simulink model "model2_cm"  (R2018b)
settings: Solver=ode8  StartTime=0.0  StopTime=Inf  FixedStep=0.01  RelTol=1e-3  EnableMultiTasking=on
StopFcn:
  | stopCallback
undefined symbols (not defined in the file): ipaddr, params, PTP
libraries: slrtlib x7, xpcutilitieslib x3, ptplib x3, xpcrtudplib x3, controllers_cl x1, find6DOF_cl x1, find6DOFSnell_cl x1, find6DOFSnellMin_cl x1, risingDebounce_ul x1, latchHigh_ul x1, manualMotorOverride_ul x1, outputCommands_ul x1
settings Model: sg_rtwmakecfg_data=_sglibc_  SimulationMode=external  Creator=mcobb  LastModifiedBy=MAE-NCSUCORE
settings SolverCC: ConcurrentTasks=on  AutoInsertRateTranBlk=on
settings DataIOCC: SaveFormat=StructureWithTime
settings OptimizationCC: BlockReduction=off  UseFloatMulNetSlope=on  EnhancedBackFolding=on  PassReuseOutputArgsThreshold=0  EfficientFloat2IntCast=on  OptimizeBlockOrder=speed  DifferentSizesBufferReuse=on  OptimizationCustomize=off
settings DebuggingCC: ParameterOverflowMsg=none  ParameterTunabilityLossMsg=error  LibraryContextMissingDiagnostic=none
settings HardwareCC: ProdBitPerPointer=32  ProdBitPerSizeT=32  ProdBitPerPtrDiffT=32  ProdLargestAtomicFloat=None  ProdWordSize=32  ProdLongLongMode=on  ProdHWDeviceType=Generic->32-bit x86 compatible
settings SFSimCC: SimUseLocalCustomCode=off  MATLABDynamicMemAlloc=off
settings RTWCC: SystemTargetFile=slrt.tlc  TemplateMakefile=slrt_default_tmf  Description=Simulink Real-Time  RTWUseLocalCustomCode=off  BuildConfiguration=Debug  CodeExecutionProfiling=on  RTWCompilerOptimization=on
settings CodeAppCC: ForceParamTrailComments=on  OperatorAnnotations=on
settings SimulinkRealTimeCC: SupportVariableSizeSignals=on  PreserveStateflowLocalDataDimensions=off  RL32LogTETModifier=off  RL32ObjectName=tg2  xPCisDefaultEnv=off  xPCTargetPCEnvName=Machine2  xPCConcurrentTasks=on

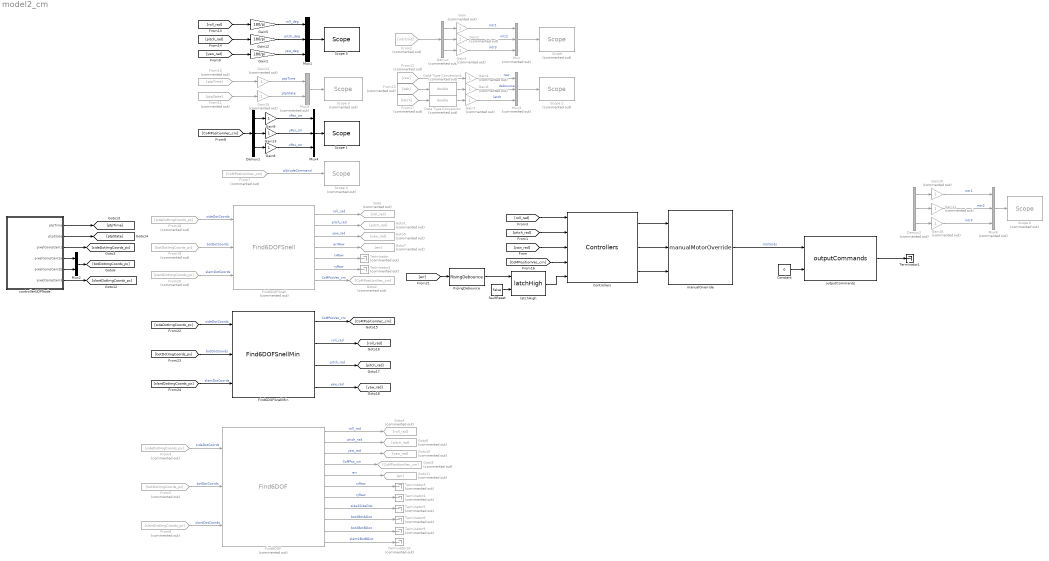
== system model2_cm ==
  Constant : Constant  Value=0
  Controllers : controllers_cl/Controllers  SystemSampleTime=-1
      link override ConstantSetpoints/AltitudeController: enable=off  kp=0.1  kd=0  timeConstant_s=0.4
      link override ConstantSetpoints/AltitudeSetpoint_cm: Value=46
      link override ConstantSetpoints/PitchController: enable=off  kp=2  kd=1  timeConstant_s=0.3
      link override ConstantSetpoints/PitchSetpoint_deg: Value=5
      link override ConstantSetpoints/RollController: enable=off  kp=2  kd=1  timeConstant_s=0.02
      link override ConstantSetpoints/RollSetpoint_deg: Value=0
  Data Type Conversion : DataTypeConversion  Commented=on  OutDataTypeStr=double
  Data Type Conversion1 : DataTypeConversion  Commented=on  OutDataTypeStr=double
  Demux : Demux  Commented=on  Outputs=3
  Demux1 : Demux  Outputs=3
  Demux2 : Demux  Commented=on  Outputs=3
  Find6DOF : find6DOF_cl/Find6DOF  Commented=on  imageDims_px=params.sideImageSize_px.Value  initialCoMPositionVec_cm=params.initCoMPosVec_cm.Value  cameraFOVAngles_deg=params.cameraFOV_deg.Value  sideEulerAngles_deg=params.sideCamEulAng_deg.Value  sideCamPositionVec_cm=params.sideCamPosVec_cm.Value  botEulerAngles_deg=params.botCamEulAng_deg.Value  botCamPositionVec_cm=params.botCamPosVec_cm.Value  slantEulerAngles_deg=params.slntCamEulAng_deg.Value  slantCamPositionVec_cm=params.slntCamPosVec_cm.Value  sideSeparation_cm=params.sideDotSepDist_cm.Value  sidePositionVecBF_cm=params.sideDotPosVec_cm.Value  bottomASeparation_cm=params.botADotSepDist_cm.Value  botAPositionVecBF_cm=params.botADotPosVec_cm.Value  bottomBSeparation_cm=params.botBDotSepDist_cm.Value  botBPositionVecBG_cm=params.botBDotPosVec_cm.Value
  Find6DOFSnell : find6DOFSnell_cl/Find6DOFSnell  Commented=on  imageDims_px=params.sideImageSize_px.Value  initialCoMPositionVec_cm=params.initCoMPosVec_cm.Value  indxOfRefVec=params.indexOfRefractionA.Value  glassThickness_cm=params.glassThickness_cm.Value  cameraFOVAngles_deg=params.cameraFOV_deg.Value  sideEulerAngles_deg=params.sideCamEulAng_deg.Value  sideCamPositionVec_cm=params.sideCamPosVec_cm.Value  sideCamDistToGlass_cm=params.sideDistancetoGlass_cm.Value  botEulerAngles_deg=params.botCamEulAng_deg.Value  botCamPositionVec_cm=params.botCamPosVec_cm.Value  botCamDistToGlass_cm=params.botDistancetoGlass_cm.Value  slantEulerAngles_deg=params.slntCamEulAng_deg.Value  slantCamPositionVec_cm=params.slntCamPosVec_cm.Value  slantCamDistToGlass_cm=params.slntDistancetoGlass_cm.Value  sideSeparation_cm=params.sideDotSepDist_cm.Value  sidePositionVecBF_cm=params.sideDotPosVec_cm.Value  bottomASeparation_cm=params.botADotSepDist_cm.Value  botAPositionVecBF_cm=params.botADotPosVec_cm.Value  bottomBSeparation_cm=params.botBDotSepDist_cm.Value  botBPositionVecBG_cm=params.botBDotPosVec_cm.Value
  Find6DOFSnellMin : find6DOFSnellMin_cl/Find6DOFSnellMin  imageDims_px=params.sideImageSize_px.Value  initialCoMPositionVec_cm=params.initCoMPosVec_cm.Value  initialEulerAngles_deg=params.initEulerAng_deg.Value  indxOfRefVec=params.indexOfRefractionA.Value  glassThickness_cm=params.glassThickness_cm.Value  cameraFOVAngles_deg=params.cameraFOV_deg.Value  sideEulerAngles_deg=params.sideCamEulAng_deg.Value  sideCamPositionVec_cm=params.sideCamPosVec_cm.Value  sideCamDistToGlass_cm=params.sideDistancetoGlass_cm.Value  botEulerAngles_deg=params.botCamEulAng_deg.Value  botCamPositionVec_cm=params.botCamPosVec_cm.Value  botCamDistToGlass_cm=params.botDistancetoGlass_cm.Value  slantEulerAngles_deg=params.slntCamEulAng_deg.Value  slantCamPositionVec_cm=params.slntCamPosVec_cm.Value  slantCamDistToGlass_cm=params.slntDistancetoGlass_cm.Value  sideSeparation_cm=params.sideDotSepDist_cm.Value  sidePositionVecBF_cm=params.sideDotPosVec_cm.Value  bottomASeparation_cm=params.botADotSepDist_cm.Value  botAPositionVecBF_cm=params.botADotPosVec_cm.Value  bottomBSeparation_cm=params.botBDotSepDist_cm.Value  botBPositionVecBF_cm=params.botBDotPosVec_cm.Value
  From10 : From  Commented=on  GotoTag=ptpTime
  From11 : From  Commented=on  GotoTag=ptpState
  From12 : From  Commented=on  GotoTag=raw
  From15 : From  Commented=on  GotoTag=deb
  From17 : From  Commented=on  GotoTag=latch
  From18 : From  Commented=on  GotoTag=sideDotImgCoords_px
  From19 : From  Commented=on  GotoTag=botDotImgCoords_px
  From2 : From  Commented=on  GotoTag=mtrCmd
  From20 : From  Commented=on  GotoTag=slantDotImgCoords_px
  From4 : From  Commented=on  GotoTag=sideDotImgCoords_px
  From5 : From  Commented=on  GotoTag=botDotImgCoords_px
  From6 : From  Commented=on  GotoTag=slantDotImgCoords_px
  From7 : From  Commented=on  GotoTag=CoMPositionVec_cm
  Gain{,2..4,6..7,10..11,14..16} (11 alike) : Gain  Commented=on
  Gain1 : Gain  Gain=180/pi
  Gain12 : Gain  Gain=180/pi
  Gain13 : Gain
  Gain5 : Gain  Gain=180/pi
  Gain8 : Gain
  Gain9 : Gain
  Goto : Goto  Commented=on  GotoTag=roll_rad
  Goto1 : Goto  Commented=on  GotoTag=pitch_rad
  Goto10 : Goto  Commented=on  GotoTag=yaw_rad
  Goto11 : Goto  Commented=on  GotoTag=err
  Goto2 : Goto  Commented=on  GotoTag=CoMPositionVec_cm
  Goto4 : Goto  Commented=on  GotoTag=roll_rad
  Goto5 : Goto  Commented=on  GotoTag=yaw_rad
  Goto7 : Goto  Commented=on  GotoTag=err
  Goto8 : Goto  Commented=on  GotoTag=pitch_rad
  Goto9 : Goto  Commented=on  GotoTag=CoMPositionVec_cm
  Mux : Mux  Commented=on  Inputs=3
  Mux1 : Mux  Inputs=3
  Mux2 : Mux  Inputs=2
  Mux3 : Mux  Commented=on  Inputs=3
  Mux4 : Mux  Inputs=3
  Mux5 : Mux  Commented=on  Inputs=2
  Mux6 : Mux  Commented=on  Inputs=3
  RisingDebounce : risingDebounce_ul/RisingDebounce  threshold=7.500000e-01  timeDelay_s=params.imagProcErrDbncTm_s.Value
  "Scope " : slrtlib/Displays and Logging/Scope   Commented=on  scopeno=3  scopetype=Target  autostart=on  viewmode=Graphical rolling  formatstr='%15.6f'  grid=on  ylimits=[0,0]  nosamples=1000  noprepostsamples=0  interleave=1  triggermode=FreeRun  triggersignal=1  trigsignalfromport=off  triggerlevel=0.0  triggerslope=Either  triggerscope=1  triggersample=0  filename=data.dat  mode=Lazy  writesize=512  autorestart=off  dynamicfilemode=off  maxwritefilesize=512*1024^2
  Scope 1 : slrtlib/Displays and Logging/Scope   scopeno=3  scopetype=Target  autostart=on  viewmode=Numerical  formatstr='%15.6f'  grid=on  ylimits=[0,0]  nosamples=10  noprepostsamples=0  interleave=1  triggermode=FreeRun  triggersignal=1  trigsignalfromport=off  triggerlevel=0.0  triggerslope=Either  triggerscope=1  triggersample=0  filename=data.dat  mode=Lazy  writesize=512  autorestart=off  dynamicfilemode=off  maxwritefilesize=512*1024^2
  Scope 2 : slrtlib/Displays and Logging/Scope   Commented=on  scopeno=1  scopetype=Target  autostart=on  viewmode=Graphical rolling  formatstr='%15.6f'  grid=on  ylimits=[-0.5,1.5]  nosamples=1000  noprepostsamples=0  interleave=1  triggermode=FreeRun  triggersignal=1  trigsignalfromport=off  triggerlevel=0.0  triggerslope=Either  triggerscope=1  triggersample=0  filename=data.dat  mode=Lazy  writesize=512  autorestart=off  dynamicfilemode=off  maxwritefilesize=512*1024^2
  Scope 3 : slrtlib/Displays and Logging/Scope   Commented=on  scopeno=4  scopetype=Target  autostart=on  viewmode=Graphical rolling  formatstr='%15.6f'  grid=on  ylimits=[-30,30]  nosamples=1000  noprepostsamples=0  interleave=1  triggermode=FreeRun  triggersignal=1  trigsignalfromport=off  triggerlevel=0.0  triggerslope=Either  triggerscope=1  triggersample=0  filename=data.dat  mode=Lazy  writesize=512  autorestart=off  dynamicfilemode=off  maxwritefilesize=512*1024^2
  Scope 4 : slrtlib/Displays and Logging/Scope   Commented=on  scopeno=4  scopetype=Target  autostart=on  viewmode=Graphical rolling  formatstr='%15.6f'  grid=on  ylimits=[-1,1]  nosamples=1000  noprepostsamples=0  interleave=1  triggermode=FreeRun  triggersignal=1  trigsignalfromport=off  triggerlevel=0.0  triggerslope=Either  triggerscope=1  triggersample=0  filename=data.dat  mode=Lazy  writesize=512  autorestart=off  dynamicfilemode=off  maxwritefilesize=512*1024^2
  Scope 5 : slrtlib/Displays and Logging/Scope   scopeno=1  scopetype=Target  autostart=on  viewmode=Numerical  formatstr='%15.6f'  grid=on  ylimits=[-45,45]  nosamples=10  noprepostsamples=0  interleave=1  triggermode=FreeRun  triggersignal=1  trigsignalfromport=off  triggerlevel=0.0  triggerslope=Either  triggerscope=1  triggersample=0  filename=data.dat  mode=Lazy  writesize=512  autorestart=off  dynamicfilemode=off  maxwritefilesize=512*1024^2
  Scope 6 : slrtlib/Displays and Logging/Scope   Commented=on  scopeno=1  scopetype=Target  autostart=on  viewmode=Numerical  formatstr='%15.6f'  grid=on  ylimits=[0,0]  nosamples=10  noprepostsamples=0  interleave=1  triggermode=FreeRun  triggersignal=1  trigsignalfromport=off  triggerlevel=0.0  triggerslope=Either  triggerscope=1  triggersample=0  filename=data.dat  mode=Lazy  writesize=512  autorestart=off  dynamicfilemode=off  maxwritefilesize=512*1024^2
  Terminator{,2..6,9..10} (8 alike) : Terminator  Commented=on
  Terminator1 : Terminator
  controllerUDPNode : Subsystem  TreatAsAtomicUnit=on  mask{sample_time=0.01, announce_interval=params.announceInterval_s.Value, sync_interval=params.syncInterval_s.Value}
      mask prompts: sample_time "Sample time (-1 for inherited)"; announce_interval "Announce interval (second):"; sync_interval "Sync interval (second):"
      mask TypeOptions sample_time: IEEE 1588 Read State/sample_time | IEEE 1588 Read Time/sample_time | IEEE 1588 Real-Time UDP/sample_time | UDP Receive Machine 3/sampleTime | UDP Receive Machine 4/sampleTime | UDP Receive Machine 5/sampleTime
      mask TypeOptions announce_interval: IEEE 1588 Real-Time UDP/announce_interval
      mask TypeOptions sync_interval: IEEE 1588 Real-Time UDP/sync_interval
  faultReset : Constant  Value=false
  latchHigh : latchHigh_ul/latchHigh  SystemSampleTime=-1
  manualOverride : manualMotorOverride_ul/manualMotorOverride  enbl=1  mtr1CmdOvrrd=0  mtr2CmdOvrrd=0  mtr3CmdOvrrd=0
  outputCommands : outputCommands_ul/outputCommands  maxVoltage=params.maxOutVltg_vlt.Value
  wires:
  controllerUDPNode/3(pixelCompCam1) -> [sideDotImgCoords_px]
  controllerUDPNode/6(pixelCompCam3) -> [slantDotImgCoords_px]
  Mux5/1 -> Scope 3/1
  From7/1 -> Scope 4/1  "altitudeCommand"
  Constant/1 -> outputCommands/2
  Mux2/1 -> [botDotImgCoords_px]
  controllerUDPNode/5(pixelCompCam2b) -> Mux2/2
  controllerUDPNode/4(pixelCompCam2a) -> Mux2/1
  Gain12/1 -> Mux1/2  "pitch_deg"
  Gain5/1 -> Mux1/1  "roll_deg"
  Mux1/1 -> Scope 5/1
  [roll_rad] -> Gain5/1
  [pitch_rad] -> Gain12/1
  [CoMPositionVec_cm] -> Demux1/1
  Gain13/1 -> Mux4/2  "yPos_cm"
  From11/1 -> Gain15/1
  From10/1 -> Gain14/1
  RisingDebounce/1 -> latchHigh/1
  outputCommands/1 -> Terminator1/1
  [yaw_rad] -> Controllers/3
  [pitch_rad] -> Controllers/2
  [roll_rad] -> Controllers/1
  Controllers/1 -> manualOverride/1
  faultReset/1 -> latchHigh/2
  [CoMPositionVec_cm] -> Controllers/4
  latchHigh/1 -> Controllers/5
  Controllers/2 -> manualOverride/2
  Controllers/3 -> manualOverride/3
  [yaw_rad] -> Gain1/1
  Gain1/1 -> Mux1/3  "yaw_deg"
  Demux/3 -> Gain3/1
  Demux/2 -> Gain2/1
  Demux/1 -> Gain/1
  Mux/1 -> "Scope "/1
  From2/1 -> Demux/1
  Gain/1 -> Mux/1  "mtr1"
  Gain2/1 -> Mux/2  "mtr2"
  Gain3/1 -> Mux/3  "mtr3"
  Mux3/1 -> Scope 2/1
  Gain6/1 -> Mux3/2  "debounce"
  Gain7/1 -> Mux3/3  "latch"
  Gain4/1 -> Mux3/1  "raw"
  From17/1 -> Data Type Conversion/1
  From15/1 -> Data Type Conversion1/1
  Data Type Conversion/1 -> Gain7/1
  Data Type Conversion1/1 -> Gain6/1
  From12/1 -> Gain4/1
  From18/1 -> Find6DOFSnell/1  "sideDotCoords"
  From19/1 -> Find6DOFSnell/2  "botDotCoords"
  From20/1 -> Find6DOFSnell/3  "slantDotCoords"
  Find6DOFSnell/1 -> Goto/1  "roll_rad"
  Find6DOFSnell/2 -> Goto1/1  "pitch_rad"
  Find6DOFSnell/3 -> Goto5/1  "yaw_rad"
  Find6DOFSnell/4 -> Goto7/1  "errRaw"
  Find6DOFSnell/7 -> Goto2/1  "CoMPosVec_cm"
  controllerUDPNode/1(ptpTime) -> [ptpTime]
  controllerUDPNode/2(ptpState) -> [ptpState]
  Find6DOFSnell/5 -> Terminator/1  "rxRaw"
  Find6DOFSnell/6 -> Terminator2/1  "ryRaw"
  [err] -> RisingDebounce/1
  Demux1/2 -> Gain13/1
  Demux1/3 -> Gain8/1
  Demux1/1 -> Gain9/1
  Mux4/1 -> Scope 1/1
  Gain9/1 -> Mux4/1  "xPos_cm"
  Gain8/1 -> Mux4/3  "zPos_cm"
  From4/1 -> Find6DOF/1  "sideDotCoords"
  From6/1 -> Find6DOF/3  "slantDotCoords"
  From5/1 -> Find6DOF/2  "botDotCoords"
  Find6DOF/1 -> Goto4/1  "roll_rad"
  Find6DOF/2 -> Goto8/1  "pitch_rad"
  Find6DOF/3 -> Goto10/1  "yaw_rad"
  Find6DOF/4 -> Goto9/1  "CoMPos_cm"
  Find6DOF/5 -> Goto11/1  "err"
  Find6DOF/6 -> Terminator3/1  "rxRaw"
  Find6DOF/7 -> Terminator4/1  "ryRaw"
  Find6DOF/11 -> Terminator10/1  "slant2BotBDist"
  Find6DOF/10 -> Terminator9/1  "bot2BotBDist"
  Find6DOF/9 -> Terminator6/1  "bot2BotADist"
  Find6DOF/8 -> Terminator5/1  "side2SideDist"
  Mux6/1 -> Scope 6/1
  Demux2/2 -> Gain11/1
  Demux2/1 -> Gain10/1
  Demux2/3 -> Gain16/1
  Gain10/1 -> Mux6/1  "mtr1"
  Gain11/1 -> Mux6/2  "mtr2"
  Gain16/1 -> Mux6/3  "mtr3"
  manualOverride/1 -> outputCommands/1  "mtrCmds"
  Gain14/1 -> Mux5/1  "ptpTime"
  Gain15/1 -> Mux5/2  "ptpState"
  [sideDotImgCoords_px] -> Find6DOFSnellMin/1  "sideDotCoords"
  [slantDotImgCoords_px] -> Find6DOFSnellMin/3  "slantDotCoords"
  [botDotImgCoords_px] -> Find6DOFSnellMin/2  "botDotCoords"
  Find6DOFSnellMin/1 -> [CoMPositionVec_cm]  "CoMPosVec_cm"
  Find6DOFSnellMin/4 -> [yaw_rad]  "yaw_rad"
  Find6DOFSnellMin/2 -> [roll_rad]  "roll_rad"
  Find6DOFSnellMin/3 -> [pitch_rad]  "pitch_rad"

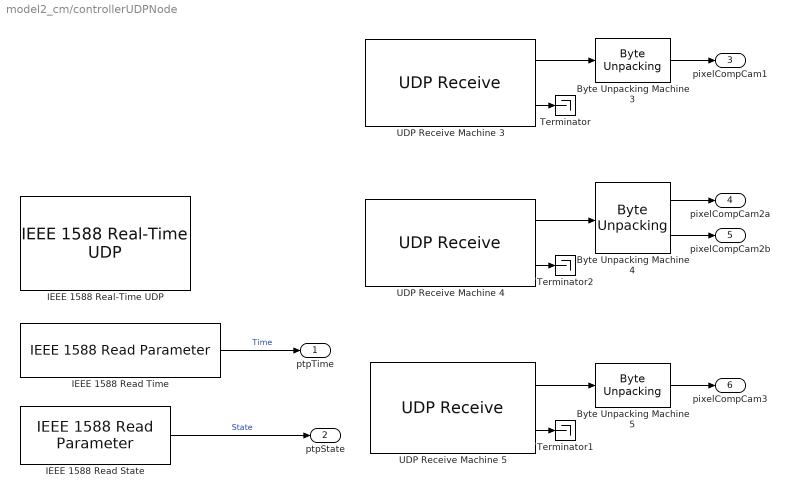
== system model2_cm/controllerUDPNode ==
  "Byte Unpacking Machine 3 " : xpcutilitieslib/Byte Unpacking   MaskUnpackedDataTypes={['double']}  MaskUnpackedDataSizes={[4]}  MaskAlignment=1
      settings: SourceProductName=Simulink Real-Time  SourceProductBaseCode=XP
  Byte Unpacking Machine 4 : xpcutilitieslib/Byte Unpacking   MaskUnpackedDataTypes={['double'],['double']}  MaskUnpackedDataSizes={[4],[4]}  MaskAlignment=1
      settings: SourceProductName=Simulink Real-Time  SourceProductBaseCode=XP
  Byte Unpacking Machine 5 : xpcutilitieslib/Byte Unpacking   MaskUnpackedDataTypes={['double']}  MaskUnpackedDataSizes={[4]}  MaskAlignment=1
      settings: SourceProductName=Simulink Real-Time  SourceProductBaseCode=XP
  IEEE 1588 Read State : ptplib/IEEE 1588 Read Parameter  Priority=1  ID=1  param=Protocol state  sample_time=sample_time  enable_read_precision=off
      settings: SourceProductName=Simulink Real-Time  SourceProductBaseCode=XP
  IEEE 1588 Read Time : ptplib/IEEE 1588 Read Parameter  Priority=1  ID=1  param=PTP time (time-of-day)  sample_time=sample_time  enable_read_precision=off
      settings: SourceProductName=Simulink Real-Time  SourceProductBaseCode=XP
  IEEE 1588 Real-Time UDP : ptplib/IEEE 1588 Real-Time UDP  Priority=0  ID=1  PciBus=2  PciSlot=0  PciFunction=0  time_inc=4000000  sample_time=sample_time  IpSource=Specify  IpAddress=30.30.30.30  SubnetMask=255.255.255.0  Gateway=0.0.0.0  Receive1=0.0.0.0  dest_ip_select=Specify  custom_dest_ip_addr=255.255.255.255  MulticastList=[ipaddr('224.0.1.129'), ipaddr('224.0.0.107')]  Multicast={macaddr('01:00:5E:00:01:81'), macaddr('01:00:5E:00:00:6B')}  time_source=Ethernet board  timescale=PTP (1970-01-01)  epoch=[1970 01 01 00]  delay_measure=Request-response  slave_only=off  enable_advanced_config=on  domain_num=0  utc_offset=35  priority1=1  clock_class=248  clock_accuracy=hex2dec('FE')  priority2=1  announce_interval=announce_interval  sync_interval=sync_interval  min_pdelay_req_interval=2  announce_receipt_timeout=30
      settings: SourceProductName=Simulink Real-Time  SourceProductBaseCode=XP
  Terminator : Terminator
  Terminator1 : Terminator
  Terminator2 : Terminator
  UDP Receive Machine 3 : xpcrtudplib/UDP Receive  ipAddressVal=30.30.30.30  localPort=8001  rcvWidth=32  rcvFmAny=off  fmAddress=30.30.30.1  rcvMulticast=off  multicastAddress={30.30.30.1, 30.30.30.2, 30.30.30.3}  maxUDPQueue=8  sampleTime=sample_time
      settings: SourceProductName=Simulink Real-Time
  UDP Receive Machine 4 : xpcrtudplib/UDP Receive  ipAddressVal=30.30.30.30  localPort=8002  rcvWidth=64  rcvFmAny=off  fmAddress=30.30.30.2  rcvMulticast=off  multicastAddress={30.30.30.1, 30.30.30.2, 30.30.30.3}  maxUDPQueue=8  sampleTime=sample_time
      settings: SourceProductName=Simulink Real-Time
  UDP Receive Machine 5 : xpcrtudplib/UDP Receive  ipAddressVal=30.30.30.30  localPort=8003  rcvWidth=32  rcvFmAny=off  fmAddress=30.30.30.3  rcvMulticast=off  multicastAddress={30.30.30.1, 30.30.30.2, 30.30.30.3}  maxUDPQueue=8  sampleTime=sample_time
      settings: SourceProductName=Simulink Real-Time
  ptpTime : Outport
  ptpState : Outport  Port=2
  pixelCompCam1 : Outport  Port=3
  pixelCompCam2a : Outport  Port=4
  pixelCompCam2b : Outport  Port=5
  pixelCompCam3 : Outport  Port=6
  wires:
  UDP Receive Machine 3/1 -> "Byte Unpacking Machine 3 "/1
  UDP Receive Machine 4/1 -> Byte Unpacking Machine 4/1
  IEEE 1588 Read Time/1 -> ptpTime/1  "Time"
  UDP Receive Machine 3/2 -> Terminator/1
  UDP Receive Machine 5/2 -> Terminator1/1
  "Byte Unpacking Machine 3 "/1 -> pixelCompCam1/1
  UDP Receive Machine 4/2 -> Terminator2/1
  Byte Unpacking Machine 5/1 -> pixelCompCam3/1
  IEEE 1588 Read State/1 -> ptpState/1  "State"
  UDP Receive Machine 5/1 -> Byte Unpacking Machine 5/1
  Byte Unpacking Machine 4/1 -> pixelCompCam2a/1
  Byte Unpacking Machine 4/2 -> pixelCompCam2b/1
